simulink model "fwv_modified"  (R2021a)
settings: Solver=ode23t  StartTime=0.0  StopTime=9  FixedStep=0.01  MaxStep=0.01  RelTol=1e-3  AbsTol=1e-3  EnableMultiTasking=on
model workspace: external: MATLAB File param.m (data not in the file)
values from neighbouring files (symbols this model uses):
  A_D = 1.5    [main.m]    (also in param.m; params.m)
  A_L = 1.8    [main.m]    (also in param.m; params.m)
  c_bar = 0.035714285714285712    (= 0.0357142857143)    [main.m]    (also in param.m = 0.0251327412287; params.m)
  C_D0 = 0.45    [main.m]    (also in param.m; params.m)
  f = 37.5    [param.m]
  ht = 4    [main.m]    (also in param.m)
  m = 2    [rbf_pid.m]
  r00 = 0.93333333333333335    (= 0.933333333333)    [main.m]    (also in param.m = 1; params.m)
  r11 = 0.48118518518518516    (= 0.481185185185)    [main.m]    (also in param.m = double(int(curv(x)*(x+1/9),0,1)); params.m)
  r22 = 0.30475061728395064    (= 0.304750617284)    [main.m]    (also in param.m = double(int(curv(x)*(x+1/9)^2,0,1)); params.m)
  r33 = 0.2185686913580247    (= 0.218568691358)    [main.m]    (also in param.m = double(int(curv(x)*(x+1/9)^3,0,1)); params.m)
  r_cp = 0.10758076225045371    (= 0.10758076225)    [main.m]    (also in param.m = Rw*r33/r22; params.m)
  rho = 1.205    [main.m]    (also in param.m; params.m)
  Rw = 0.15    [main.m]    (also in param.m = 0.075; params.m)
  z00 = 1.0017777777777779    (= 1.00177777778)    [main.m]    (also in param.m = double(int(curv(x)^2,0,1)); params.m)
  z11 = 0.48491851851851853    (= 0.484918518519)    [main.m]    (also in param.m = double(int(curv(x)^2*(x+1/9),0,1)); params.m)
  z22 = 0.28785382716049385    (= 0.28785382716)    [main.m]    (also in param.m = double(int(curv(x)^2*(x+1/9)^2,0,1)); params.m)
  zrd = 1.2933386666666666    (= 1.29333866667)    [main.m]    (also in param.m = double(int(curv(x)^4,0,1)); params.m)
undefined symbols (not defined in the file or in its folder): X, Y, Z
libraries: sm_lib x63, nesl_utility x41, vrlib x3, slpidlib x2, simulink x1
(part 1 of 3)
settings Model: NumberOfSteps=10  PacingRate=1000  OrderedModelArguments=off  Creator=jeff  LastModifiedBy=jeff
settings SolverCC: AutoScaleAbsTol=off  ZeroCrossAlgorithm=Adaptive  SolverResetMethod=Robust
settings DataIOCC: LimitDataPoints=on  MaxDataPoints=10000  DSMLogging=off  InspectSignalLogs=on  SaveTime=off  ReturnWorkspaceOutputs=off
settings OptimizationCC: LifeSpan=inf
settings DebuggingCC: AllowSymbolicDim=off  SFUnexpectedBacktrackingDiag=warning  SFNoUnconditionalDefaultTransitionDiag=warning  SFExecutionAtInitializationDiag=none  SFMachineParentedDataDiag=warning  ArithmeticOperatorsInVariantConditions=warning
settings ModelReferenceCC: ModelReferenceMinAlgLoopOccurrences=on
settings SFSimCC: SimUseLocalCustomCode=off  CustomCodeUndefinedFunction=UseInterfaceOnly
settings RTWCC: RTWUseLocalCustomCode=off
settings CodeAppCC: StateflowObjectComments=on
settings GRTTargetCC: TargetLangStandard=C89/C90 (ANSI)
settings ConfigComp: CovMetricSettings=dw  CovSaveCumulativeToWorkspaceVar=on  CovSaveSingleToWorkspaceVar=on  CovExternalEMLEnable=off  CovSFcnEnable=off
settings SimscapeCC: SimscapeLogType=all  SimscapeLogSimulationStatistics=on  SimscapeLogDataHistory=10000
settings ExplorerConfigSet: InternalSimMechanicsExplorerSettings="<ExplorerConfiguration><canonicalview>default</canonicalview><AnimationSetting><BasePlaybackSpeed>1.0</BasePlaybackSpeed><PlaybackSpeedFactor>1.0</PlaybackSpeedFactor></AnimationSetting><TilePanel><TileInfo><Tiles Columns=\"2\" Count=\"4\" Rows=\"2\"><Column Weight=\"0.5\"/><Column Weight=\"0.5\"/><Row Weight=\"0.4982\"/><Row Weight=\"0.5018\"/><Tile Height=\"1\" Width=\"1\" X=\"0\" Y=\"0\"/><Tile Height=\"1\" Width=\"1\" X=\"0\" Y=\"1\"/><Tile Height=\"1\" Width=\"1\" X=\"1\" Y=\"0\"/><Tile Height=\"1\" Width=\"1\" X=\"1\" Y=\"1\"/></Tiles></TileInfo><SceneInfo><SceneViewer><BGColor><R>0.60000002384185791</R><G>0.60000002384185791</G><B>0.60000002384185791</B></BGColor><Camera><DoPerspective>off</DoPerspective><Position><X>1.52276591336431011e-07</X><Y>-15.7283506478538051</Y><Z>0.997276938595945239</Z></Position><Center><X>1.52276591336431011e-07</X><Y>8.81149515574719544e-08</Y><Z>0.997276938595945239</Z></Center><Up><X>0</X><Y>-0</Y><Z>1</Z></Up><ViewLimDist>1</ViewLimDist><YLim>4.13867069486404926</YLim><XLim>10.3000000000000007</XLim></Camera></SceneViewer><SceneViewer><BGColor><R>0.60000002384185791</R><G>0.60000002384185791</G><B>0.60000002384185791</B></BGColor><Camera><DoPerspective>off</DoPerspective><Position><X>1.52276591336431011e-07</X><Y>-4.72670020457144346e-07</Y><Z>14.1965844691727394</Z></Position><Center><X>1.52276591336431011e-07</X><Y>-4.72670020457144346e-07</Y><Z>0.997276770136494406</Z></Center><Up><X>0</X><Y>1</Y><Z>-0</Z></Up><ViewLimDist>1</ViewLimDist><YLim>10.3000000000000007</YLim><XLim>25.4425373134328368</XLim></Camera></SceneViewer><SceneViewer><BGColor><R>0.60000002384185791</R><G>0.60000002384185791</G><B>0.60000002384185791</B></BGColor><Camera><DoPerspective>off</DoPerspective><Position><X>15.7283506450403667</X><Y>-4.72670020457144346e-07</Y><Z>0.997277415433075021</Z></Position><Center><X>1.16597679067353965e-06</X><Y>-4.72670020457144346e-07</Y><Z>0.997277415433075021</Z></Center><Up><X>-0</X><Y>0</Y><Z>1</Z></Up><ViewLimDist>1</ViewLimDist><YLim>4.13867069486404926</YLim><XLim>10.3000000000000007</XLim></Camera></SceneViewer><SceneViewer><BGColor><R>0.60000002384185791</R><G>0.60000002384185791</G><B>0.60000002384185791</B></BGColor><Camera><DoPerspective>on</DoPerspective><Position><X>2.15185180954951205</X><Y>2.000061471445302</Y><Z>2.10008566610887026</Z></Position><Center><X>2.00185180954951214</X><Y>2.000061471445302</Y><Z>2.00008566610887017</Z></Center><Up><X>0</X><Y>-3.08148791101957736e-33</Y><Z>1</Z></Up><ViewLimDist>1</ViewLimDist><YLim>0.466307658154998583</YLim><XLim>1.15184951380078004</XLim></Camera></SceneViewer></SceneInfo></TilePanel><MechEditorPanel><Cameras><Camera><Id>Camera1</Id><Value><Name>Camera1</Name><NativeCamera><PositionTrackingFeature>FWV.camera.camera_Frame.R</PositionTrackingFeature><CenterTrackingFeature>FWV.camera.C</CenterTrackingFeature><UpVectorTrackingFeature>FWV.camera.C</UpVectorTrackingFeature><CenterTrackingOrigin>on</CenterTrackingOrigin><UpVectorTrackingDirection>+Z</UpVectorTrackingDirection></NativeCamera></Value></Camera></Cameras><GfxPanelCameraMap><MapElement CameraMLId=\"Camera1\" GfxPanelIndex=\"3\"/></GfxPanelCameraMap><VideoCreator><PlaybackSpeedRatio>1.0</PlaybackSpeedRatio><FrameRate>30</FrameRate><VideoFormat>Motion JPEG AVI</VideoFormat><FrameSize>auto</FrameSize></VideoCreator></MechEditorPanel></ExplorerConfiguration>"

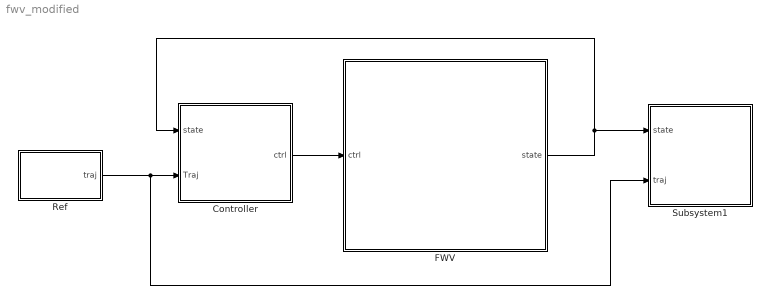
== system fwv_modified ==
  Controller : Subsystem
  FWV : Subsystem  mask{rho_w=800, m_t=20, stif_stk=1e-2, stif_rot=5e-3, damp_rot=0, stif_m=1e2, damp_m=1e2, z0=0, p0=0, q0=0, r0=0}
      mask prompts: z0 "initial height"; p0 "initial roll(deg)"; q0 "initial pitch(deg)"; r0 "initial yaw(deg)"
      mask Display: image('Images/fwv.png');
  Ref : Subsystem
  Subsystem1 : Subsystem
  wires:
  Ref/1(traj) -> Subsystem1/2(traj), Controller/2(Traj)
  Controller/1(ctrl) -> FWV/1(ctrl)
  FWV/1(state) -> Controller/1(state), Subsystem1/1(state)

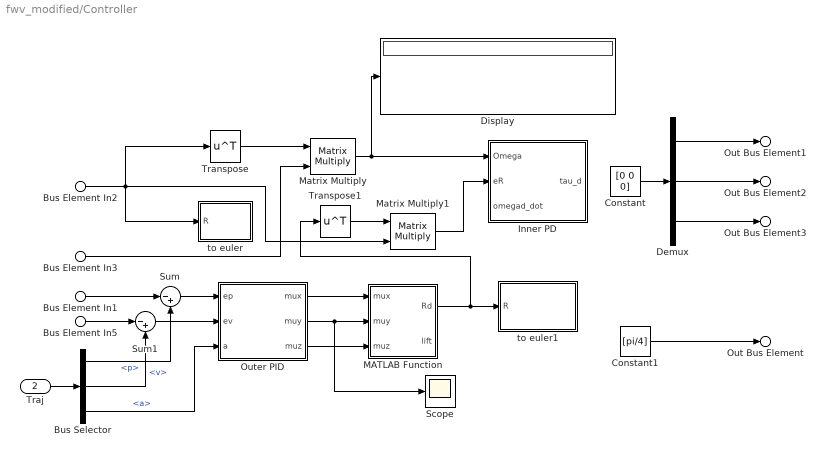
== system fwv_modified/Controller ==
  Bus Element In1 : Inport  PortName=state  Element=pose.p
  Bus Element In2 : Inport  PortName=state  Element=pose.R
  Bus Element In3 : Inport  PortName=state  Element=pose.Rd
  Bus Element In5 : Inport  PortName=state  Element=pose.v
  Traj : Inport  Port=2
  Bus Selector : BusSelector  OutputSignals=p,v,a
  Constant : Constant  Value=[0 0 0]
  Constant1 : Constant  Value=[pi/4]
  Demux : Demux  Outputs=3
  Display : Display
  Inner PD : Subsystem
  MATLAB Function : MATLAB Function  TreatAsAtomicUnit=on
  Matrix Multiply : Product  Multiplication=Matrix(*)
  Matrix Multiply1 : Product  Multiplication=Matrix(*)
  Outer PID : Subsystem
  Scope : Scope
  Sum : Sum  Inputs=|-+
  Sum1 : Sum  Inputs=|-+
  Transpose : Math  Operator=transpose  SaturateOnIntegerOverflow=on
  Transpose1 : Math  Operator=transpose  SaturateOnIntegerOverflow=on
  to euler : Subsystem
  to euler1 : Subsystem
  Out Bus Element : Outport  PortName=ctrl  Element=amp_mean
  Out Bus Element1 : Outport  PortName=ctrl  Element=amp_diff
  Out Bus Element2 : Outport  PortName=ctrl  Element=bias
  Out Bus Element3 : Outport  PortName=ctrl  Element=offset
  wires:
  Bus Element In1/1 -> Sum/1
  Traj/1 -> Bus Selector/1
  Bus Selector/1 -> Sum/2  "<p>"
  Demux/1 -> Out Bus Element1/1
  Demux/2 -> Out Bus Element2/1
  Demux/3 -> Out Bus Element3/1
  Bus Element In2/1 -> Matrix Multiply1/2, to euler/1(R), Transpose/1
  Sum/1 -> Outer PID/1(ep)
  Matrix Multiply1/1 -> Inner PD/2(eR)
  Matrix Multiply/1 -> Display/1, Inner PD/1(Omega)
  Transpose/1 -> Matrix Multiply/1
  Bus Element In3/1 -> Matrix Multiply/2
  Outer PID/1(mux) -> MATLAB Function/1(mux)
  Outer PID/2(muy) -> Scope/1, MATLAB Function/2(muy)
  Outer PID/3(muz) -> MATLAB Function/3(muz)
  Transpose1/1 -> Matrix Multiply1/1
  MATLAB Function/1(Rd) -> Transpose1/1, to euler1/1(R)
  Bus Element In5/1 -> Sum1/1
  Sum1/1 -> Outer PID/2(ev)
  Bus Selector/2 -> Sum1/2  "<v>"
  Bus Selector/3 -> Outer PID/3(a)  "<a>"
  Constant/1 -> Demux/1
  Constant1/1 -> Out Bus Element/1

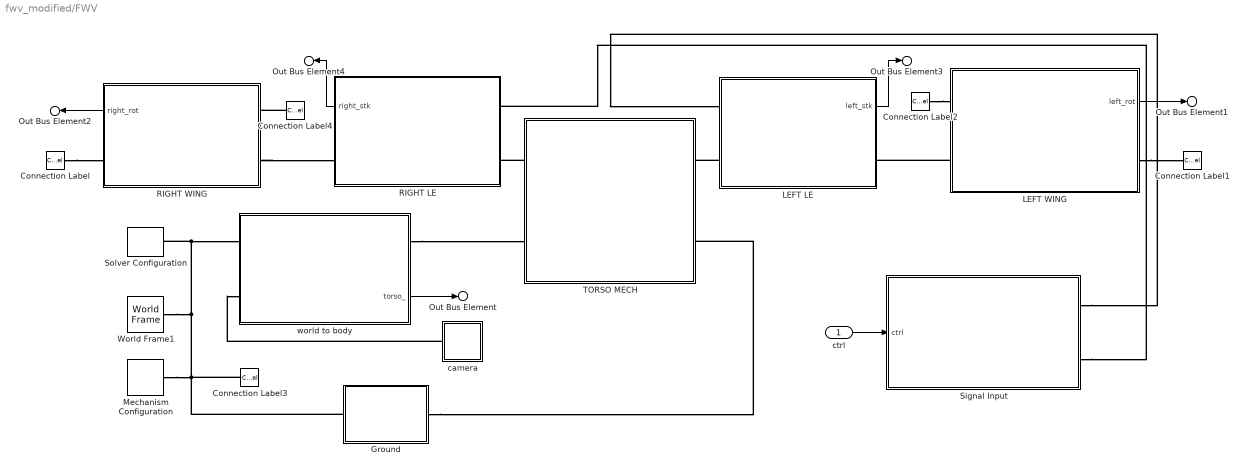
== system fwv_modified/FWV ==
  ctrl : Inport
  Connection Label : ConnectionLabel  Label=CP_R
  Connection Label1 : ConnectionLabel  Label=CP_L
  Connection Label2 : ConnectionLabel  Label=W
  Connection Label3 : ConnectionLabel  Label=W
  Connection Label4 : ConnectionLabel  Label=W
  Ground : Subsystem
  LEFT LE : Subsystem
      mask Display: image('Images/lle.png'); % Use "Edit Image" on toolstrip to change.
  LEFT WING : Subsystem
      mask Display: image('Images/lwing.png'); % Use "Edit Image" on toolstrip to change.
  Mechanism Configuration : sm_lib/Utilities/Mechanism Configuration  UniformGravity=Constant  GravityVector=[0 0 -9.80665]  GravityVectorUnits=m/s^2  GravityUnits=m/s^2  LinearizationDelta=0.001  JointModeTransitionNonlinearIterations=2
  RIGHT LE : Subsystem
      settings: PortSchema="{\"entries\":[{\"content\":{\"sides\":[{\"content\":{\"connectorIds\":[\"Out1\",\"LConn1\"]},\"type\":\"ConnectorPlacement.EquallySpacedRectSide\",\"uuid\":\"e80f0529-82a8-4e91-8f70-1f5fff48efb0\"},{\"content\":{\"connectorIds\":[\"RConn1\",\"RConn2\"],\"side\":\"RIGHT\"},\"type\":\"ConnectorPlacement.EquallySpacedRectSide\",\"uuid\":\"c7e3ee7d-7bee-46da-b210-768e5832b89d\"},{\"content\":{\"connectorIds\":[],\"side\":\"TOP\"},\"type\":\"ConnectorPlacement.EquallySpacedRectSide\",\"uuid\":\"680cbd67-40e5-4a58-a196-f2062cf587c7\"}]},\"type\":\"ConnectorPlacement.EquallySpacedConnector\",\"uuid\":\"7cb1a5ec-7352-40bf-9e6c-a29cba360f94\"}],\"packageUris\":[\"http://schema.mathworks.com/mf0/Connector/R2020b\"],\"version\":\"1.0\"}"
      mask Display: image('Images/rle.png'); % Use "Edit Image" on toolstrip to change.
  RIGHT WING : Subsystem
      mask Display: image('Images/rwing.png'); % Use "Edit Image" on toolstrip to change.
  Signal Input : Subsystem
  Solver Configuration : nesl_utility/Solver Configuration  PhysicalDomain=network_engine_domain  SubClassName=solver  LeftPortType=input  RightPortType=generic  Tones=[]  Harmonics=[]  SimulateNoise=off  Profile=off  UseLocalSampling=off  EnableSwitchedLinearOptims=on  FrequencyDomain=off  UseCCode=off  RelTol=0.001  AbsTol=1e-06  MinStep=1e-09  ToWorkspace=off  RevertToSquareIcSolve=off  NumHomotopyIterations=100  PhasorMode=off  PhasorModeNumHarmonics=1  DoDC=off  ResidualTolerance=1e-09  UseLocalSolver=off  LocalSolverChoice=NE_BACKWARD_EULER_ADVANCER  LocalSolverSampleTime=0.001  DoFixedCost=off  MaxNonlinIter=3  MaxModeIter=2  ComputeImpulses=off  ImpulseIterations=2  LinearAlgebra=Sparse  EquationFormulation=NE_TIME_EF  DelaysMemoryBudget=1024  AutomaticFiltering=on  FilteringTimeConstant=0.001  PartitionStorageMethod=AS_NEEDED  PartitionMemoryBudget=1024  PartitionMethod=FAST
      settings: SourceProductBaseCode=PW,SS
  TORSO MECH : Subsystem  mask{mu0=0, mu1=0}
      mask Display: image('Images/torso.png'); % Use "Edit Image" on toolstrip to change.
  World Frame1 : sm_lib/Frames and Transforms/World Frame
  camera : Subsystem
  world to body : Subsystem
      settings: PortSchema="{\"entries\":[{\"content\":{\"sides\":[{\"content\":{\"connectorIds\":[\"LConn1\",\"LConn2\"]},\"type\":\"ConnectorPlacement.EquallySpacedRectSide\",\"uuid\":\"67e08b7d-27a7-478e-aa2b-0a29cfb8c4ba\"},{\"content\":{\"connectorIds\":[\"RConn1\",\"Out1\"],\"side\":\"RIGHT\"},\"type\":\"ConnectorPlacement.EquallySpacedRectSide\",\"uuid\":\"af848fd7-c404-4734-a34f-7cffff1411b1\"},{\"content\":{\"connectorIds\":[],\"side\":\"TOP\"},\"type\":\"ConnectorPlacement.EquallySpacedRectSide\",\"uuid\":\"40c86437-2469-4d2e-8b61-7b3eee85e893\"}]},\"type\":\"ConnectorPlacement.EquallySpacedConnector\",\"uuid\":\"cd10b607-3f85-4cd2-a6c3-0d07bf2597bd\"}],\"packageUris\":[\"http://schema.mathworks.com/mf0/Connector/R2020b\"],\"version\":\"1.0\"}"
  Out Bus Element : Outport  PortName=state  Element=pose
  Out Bus Element3 : Outport  PortName=state  Element=left_stk
  Out Bus Element1 : Outport  PortName=state  Element=left_rot
  Out Bus Element4 : Outport  PortName=state  Element=right_stk
  Out Bus Element2 : Outport  PortName=state  Element=right_rot
  wires:
  LEFT WING/1(left_rot) -> Out Bus Element1/1
  RIGHT WING/1(right_rot) -> Out Bus Element2/1
  world to body/1(torso_) -> Out Bus Element/1
  ctrl/1 -> Signal Input/1(ctrl)
  LEFT LE/1(left_stk) -> Out Bus Element3/1
  RIGHT LE/1(right_stk) -> Out Bus Element4/1
  connections:
  LEFT LE/LConn2 -- TORSO MECH/RConn1
  TORSO MECH/LConn1 -- RIGHT LE/RConn2
  Mechanism Configuration/RConn1 -- Connection Label3/LConn1 -- Ground/LConn1 -- world to body/LConn1 -- Solver Configuration/RConn1 -- World Frame1/RConn1
  world to body/RConn1 -- TORSO MECH/LConn2
  camera/LConn1 -- world to body/LConn2
  Ground/RConn1 -- TORSO MECH/RConn2
  Connection Label/LConn1 -- RIGHT WING/RConn1
  LEFT WING/RConn1 -- Connection Label1/LConn1
  LEFT WING/LConn2 -- LEFT LE/RConn1
  RIGHT WING/LConn2 -- RIGHT LE/LConn1
  Connection Label2/LConn1 -- LEFT WING/LConn1
  Connection Label4/LConn1 -- RIGHT WING/LConn1
  Signal Input/RConn1 -- LEFT LE/LConn1
  Signal Input/RConn2 -- RIGHT LE/RConn1

== system fwv_modified/Ref ==
  Bus Creator : BusCreator  Inputs=3
  Clock : Clock
  Mux1 : Mux  Inputs=3
  p,pdot,pddot : MATLAB Function  TreatAsAtomicUnit=on
  pitch : Step  Time=0  After=2  SampleTime=0  ZeroCross=off
  roll : Step  Time=0  After=0  SampleTime=0  ZeroCross=off
  yaw : Step  Time=0  After=0  SampleTime=0  ZeroCross=off
  traj : Outport
  wires:
  roll/1 -> Mux1/1
  yaw/1 -> Mux1/3
  pitch/1 -> Mux1/2
  Bus Creator/1 -> traj/1
  p,pdot,pddot/2(v) -> Bus Creator/2  "v"
  p,pdot,pddot/3(a) -> Bus Creator/3  "a"
  Clock/1 -> p,pdot,pddot/1(t)
  p,pdot,pddot/1(p) -> Bus Creator/1  "p"

== system fwv_modified/Subsystem1 ==
  Bus Element In1 : Inport  PortName=state  Element=pose.p
  Bus Element In : Inport  Port=2  PortName=traj  Element=p
  Demux : Demux  Outputs=3
  Terminator : Terminator
  To Workspace : ToWorkspace  VariableName=p  SampleTime=-1
      settings: Save2DSignal=2-D array (concatenate along first dimension)
  To Workspace1 : ToWorkspace  VariableName=pd  SampleTime=-1
      settings: Save2DSignal=2-D array (concatenate along first dimension)
  XY Graph : simulink/Sinks/XY Graph  xmin=-2  xmax=1  ymin=-1  ymax=1  st=-1
  wires:
  Bus Element In1/1 -> To Workspace/1, Demux/1
  Demux/3 -> Terminator/1
  Demux/1 -> XY Graph/1
  Demux/2 -> XY Graph/2
  Bus Element In/1 -> To Workspace1/1

== system fwv_modified/Controller/Inner PD ==
  Omega : Inport
  eR : Inport  Port=2
  omegad_dot : Inport  Port=3
  Add : Sum  Inputs=-|-+
  Display : Display
  Display1 : Display
  Kd : Constant  Value=[d1,0,0;0,d2,0;0,0,d3]  mask{d1=0.02, d2=0.2, d3=0.02}
  Kp : Constant  Value=[p1,0,0;0,p2,0;0,0,p3]  mask{p1=0.3, p2=0.5, p3=0}
  Product : Product  Multiplication=Matrix(*)
  Product1 : Product  Multiplication=Matrix(*)
  Scope : Scope
  get D : Subsystem
  get P : Subsystem
  to euler1 : Subsystem
  tau_d : Outport
  wires:
  eR/1 -> to euler1/1(R), Display1/1, get P/1(eR)
  Omega/1 -> get D/1(In1)
  Kp/1 -> Product/1
  get P/1(Out) -> Product/2
  Add/1 -> tau_d/1
  Product1/1 -> Add/2
  Kd/1 -> Product1/1
  Product/1 -> Scope/1, Add/1
  get D/1(omega) -> Display/1, Product1/2
  omegad_dot/1 -> Add/3

== system fwv_modified/Controller/Outer PID ==
  ep : Inport
  ev : Inport  Port=2
  a : Inport  Port=3
  Demux : Demux  Outputs=3
  Demux1 : Demux  Outputs=3
  Demux2 : Demux  Outputs=3
  x PID : slpidlib/PID Controller  Commented=on  Controller=PID  Form=Parallel  TimeDomain=Continuous-time  UseExternalTs=off  SampleTime=-1  IntegratorMethod=Forward Euler  FilterMethod=Forward Euler  ControllerParametersSource=internal  P=0.5  I=0  D=0.1  UseFilter=on  N=25  TunerSelectOption=Transfer Function Based (PID Tuner App)  InitialConditionSource=internal  InitialConditionForIntegrator=0  InitialConditionForFilter=0  DifferentiatorICPrevScaledInput=0  ExternalReset=none  TrackingMode=off  Kt=1  LimitOutput=off  SatLimitsSource=internal  UpperSaturationLimit=0.5  LowerSaturationLimit=-0.5  LinearizeAsGain=on  AntiWindupMode=none  Kb=1  POutMin=[]  POutMax=[]  IOutMin=[]  IOutMax=[]  DOutMin=[]  DOutMax=[]  NOutMin=[]  NOutMax=[]  SumOutDataTypeStr=double  SumOutMin=[]  SumOutMax=[]  SaturationOutMin=[]  SaturationOutMax=[]  PParamMin=[]  PParamMax=[]  IParamMin=[]  IParamMax=[]  DParamMin=[]  DParamMax=[]  NParamMin=[]  NParamMax=[]  KbParamMin=[]  KbParamMax=[]  KtParamMin=[]  KtParamMax=[]  KbOutMin=[]  KbOutMax=[]  KtOutMin=[]  KtOutMax=[]  IntegratorOutMin=[]  IntegratorOutMax=[]  FilterOutMin=[]  FilterOutMax=[]  SumI1OutMin=[]  SumI1OutMax=[]  SumI2OutMin=[]  SumI2OutMax=[]  SumI3OutMin=[]  SumI3OutMax=[]  SumI4OutMin=[]  SumI4OutMax=[]  SumDOutMin=[]  SumDOutMax=[]  DifferentiatorOutMin=[]  DifferentiatorOutMax=[]  FilterDiffOutCoefMin=[]  FilterDiffOutCoefMax=[]  ReciprocalOutMin=[]  ReciprocalOutMax=[]  SumDenOutMin=[]  SumDenOutMax=[]  SumNumOutMin=[]  SumNumOutMax=[]  DivideOutMin=[]  DivideOutMax=[]  UdiffTsProdOutMin=[]  UdiffTsProdOutMax=[]  NTsProdOutMin=[]  NTsProdOutMax=[]  UintegralTsProdOutMin=[]  UintegralTsProdOutMax=[]  UngainTsProdOutMin=[]  UngainTsProdOutMax=[]  IntegratorContinuousStateAttributes=''  IntegratorStateMustResolveToSignalObject=off  IntegratorRTWStateStorageClass=Auto  FilterContinuousStateAttributes=''  FilterStateMustResolveToSignalObject=off  FilterRTWStateStorageClass=Auto  ParallelPVariant=InternalParameters  IdealPVariant=Disabled  IVariant=InternalParameters  DVariant=InternalParameters  IntegratorVariant=Continuous  SatVariant=Disabled  AWVariant=Passthrough  PCopyVariant=Disabled  TRVariant=Disabled  FdbkBlocksVariant=Forward  IdealPFdbkVariant=Disabled  SatFdbkVariant=Disabled  DerivativeFilterVariant=ContFilter  NVariant=InternalParameters  NCopyVariant=Disabled  FilterICVariant=InternalICsFilter  IntegratorICVariant=InternalICs  ExternalResetVariant=Disabled  TRSumVariant=Passthrough  SumFdbkVariant=Disabled  SumVariant=Sum_PID  TsampFilterVariant=InternalTs  TsampNgainVariant=Passthrough  TsampIntegralVariant=Passthrough  ExternalSaturationOutDataTypeStr=Inherit: Same as second input
  x PID1 : Subsystem  mask{Kp=0, Ki=0, Kd=0}
  y PID : slpidlib/PID Controller  Commented=on  Controller=PID  Form=Parallel  TimeDomain=Continuous-time  UseExternalTs=off  SampleTime=-1  IntegratorMethod=Forward Euler  FilterMethod=Forward Euler  ControllerParametersSource=internal  P=0.3  I=0  D=0.3  UseFilter=on  N=25  TunerSelectOption=Transfer Function Based (PID Tuner App)  InitialConditionSource=internal  InitialConditionForIntegrator=0  InitialConditionForFilter=0  DifferentiatorICPrevScaledInput=0  ExternalReset=none  TrackingMode=off  Kt=1  LimitOutput=off  SatLimitsSource=internal  UpperSaturationLimit=0.5  LowerSaturationLimit=-0.5  LinearizeAsGain=on  AntiWindupMode=none  Kb=1  POutMin=[]  POutMax=[]  IOutMin=[]  IOutMax=[]  DOutMin=[]  DOutMax=[]  NOutMin=[]  NOutMax=[]  SumOutMin=[]  SumOutMax=[]  SaturationOutMin=[]  SaturationOutMax=[]  PParamMin=[]  PParamMax=[]  IParamMin=[]  IParamMax=[]  DParamMin=[]  DParamMax=[]  NParamMin=[]  NParamMax=[]  KbParamMin=[]  KbParamMax=[]  KtParamMin=[]  KtParamMax=[]  KbOutMin=[]  KbOutMax=[]  KtOutMin=[]  KtOutMax=[]  IntegratorOutMin=[]  IntegratorOutMax=[]  FilterOutMin=[]  FilterOutMax=[]  SumI1OutMin=[]  SumI1OutMax=[]  SumI2OutMin=[]  SumI2OutMax=[]  SumI3OutMin=[]  SumI3OutMax=[]  SumI4OutMin=[]  SumI4OutMax=[]  SumDOutMin=[]  SumDOutMax=[]  DifferentiatorOutMin=[]  DifferentiatorOutMax=[]  FilterDiffOutCoefMin=[]  FilterDiffOutCoefMax=[]  ReciprocalOutMin=[]  ReciprocalOutMax=[]  SumDenOutMin=[]  SumDenOutMax=[]  SumNumOutMin=[]  SumNumOutMax=[]  DivideOutMin=[]  DivideOutMax=[]  UdiffTsProdOutMin=[]  UdiffTsProdOutMax=[]  NTsProdOutMin=[]  NTsProdOutMax=[]  UintegralTsProdOutMin=[]  UintegralTsProdOutMax=[]  UngainTsProdOutMin=[]  UngainTsProdOutMax=[]  IntegratorContinuousStateAttributes=''  IntegratorStateMustResolveToSignalObject=off  IntegratorRTWStateStorageClass=Auto  FilterContinuousStateAttributes=''  FilterStateMustResolveToSignalObject=off  FilterRTWStateStorageClass=Auto  ParallelPVariant=InternalParameters  IdealPVariant=Disabled  IVariant=InternalParameters  DVariant=InternalParameters  IntegratorVariant=Continuous  SatVariant=Disabled  AWVariant=Passthrough  PCopyVariant=Disabled  TRVariant=Disabled  FdbkBlocksVariant=Forward  IdealPFdbkVariant=Disabled  SatFdbkVariant=Disabled  DerivativeFilterVariant=ContFilter  NVariant=InternalParameters  NCopyVariant=Disabled  FilterICVariant=InternalICsFilter  IntegratorICVariant=InternalICs  ExternalResetVariant=Disabled  TRSumVariant=Passthrough  SumFdbkVariant=Disabled  SumVariant=Sum_PID  TsampFilterVariant=InternalTs  TsampNgainVariant=Passthrough  TsampIntegralVariant=Passthrough  ExternalSaturationOutDataTypeStr=Inherit: Same as second input
  y PID1 : Subsystem  mask{Kp=0, Ki=0, Kd=0}
  z PID1 : Subsystem  mask{Kp=50, Ki=40, Kd=20}
  mux : Outport
  muy : Outport  Port=2
  muz : Outport  Port=3
  wires:
  ep/1 -> Demux/1
  x PID1/1(Out1) -> mux/1
  y PID1/1(Out1) -> muy/1
  z PID1/1(Out1) -> muz/1
  a/1 -> Demux2/1
  Demux1/2 -> y PID1/2(In2)
  Demux2/3 -> z PID1/3(In3)
  Demux2/2 -> y PID1/3(In3)
  Demux1/1 -> x PID1/2(In2)
  Demux1/3 -> z PID1/2(In2)
  Demux/3 -> z PID1/1(In1)
  Demux2/1 -> x PID1/3(In3)
  Demux/1 -> x PID1/1(In1)
  Demux/2 -> y PID1/1(In1)
  ev/1 -> Demux1/1

== system fwv_modified/Controller/to euler ==
  R : Inport
  Mux : Mux  Inputs=3
  R to X-Y-Z Extrinsic : Subsystem  mask(Rotation Matrix to X-Y-Z Extrinsic){}
      mask help: Computes roll / pitch / yaw values assuming they correspond to X, Y, and Z rotations, applied in that order and using extrinsic rotations (rotations applied about the fixed axes of the base frame). Does not handle case where Y (pitch) rotation is +/-90 degrees.
  Terminator : Terminator
  rad2deg : Gain  Gain=180/pi
  wires:
  R/1 -> R to X-Y-Z Extrinsic/1(R)
  R to X-Y-Z Extrinsic/2(pitch) -> Mux/2
  Mux/1 -> rad2deg/1
  rad2deg/1 -> Terminator/1
  R to X-Y-Z Extrinsic/1(roll) -> Mux/1
  R to X-Y-Z Extrinsic/3(yaw) -> Mux/3

== system fwv_modified/Controller/to euler1 ==
  R : Inport
  Mux : Mux  Inputs=3
  R to X-Y-Z Extrinsic : Subsystem  mask(Rotation Matrix to X-Y-Z Extrinsic){}
      mask help: Computes roll / pitch / yaw values assuming they correspond to X, Y, and Z rotations, applied in that order and using extrinsic rotations (rotations applied about the fixed axes of the base frame). Does not handle case where Y (pitch) rotation is +/-90 degrees.
  Terminator : Terminator
  rad2deg : Gain  Gain=180/pi
  wires:
  rad2deg/1 -> Terminator/1
  R/1 -> R to X-Y-Z Extrinsic/1(R)
  Mux/1 -> rad2deg/1
  R to X-Y-Z Extrinsic/3(yaw) -> Mux/3
  R to X-Y-Z Extrinsic/1(roll) -> Mux/1
  R to X-Y-Z Extrinsic/2(pitch) -> Mux/2

== system fwv_modified/FWV/Ground ==
  Cylindrical Solid : sm_lib/Body Elements/Cylindrical Solid  GraphicAmbientColor=[0.15 0.15 0.15 1.0]  BasedOnType=Mass  CenterOfMass=[0 0 0]  CenterOfMassUnits=m  GraphicDiffuseColor=[1.0 0.2 0.4]  CylinderLength=1  CylinderLengthUnits=mm  CylinderRadius=10  CylinderRadiusUnits=m  Density=1000  DensityUnits=kg/m^3  DoExposeReferenceFrame=off  GraphicEmissiveColor=[0.0 0.0 0.0 1.0]  ExportEntireGeometry=on  SerializedFrames=<Frames><Frame><Id>Frame1</Id><Value><Name>F1</Name><Origin><Source>GeometricFeature</Source><FeatureName>top surface</FeatureName></Origin><PrimaryAxis><DefinedDirection>+Z</DefinedDirection><Source>ReferenceFrame</Source><SourceDirection>+Z</SourceDirection><FeatureName></FeatureName></PrimaryAxis><SecondaryAxis><DefinedDirection>+X</DefinedDirection><Source>ReferenceFrame</Source><SourceDirection>+X</SourceDirection><FeatureName></FeatureName></SecondaryAxis></Value></Frame></Frames>  MarkerShape=Sphere  MarkerSize=10  GraphicType=FromGeometry  InertiaType=Custom  Mass=0  MassUnits=kg  MomentsOfInertia=[1 1 1]  MomentsOfInertiaUnits=kg*m^2  GraphicOpacity=1.0  ProductsOfInertia=[0 0 0]  ProductsOfInertiaUnits=kg*m^2  GraphicShininess=75  GraphicSpecularColor=[0.5 0.5 0.5 1.0]  GraphicVisPropType=SimpleVisualProperties
  Rigid Transform : sm_lib/Frames and Transforms/Rigid Transform  TranslationMethod=StandardAxis  TranslationStandardOffset=5  TranslationLengthUnit=cm  TranslationStandardAxis=-Z  TranslationCartesianOffset=[0 0 0]  TranslationROffset=0  TranslationROffsetUnits=m  TranslationZOffset=0  TranslationZOffsetUnits=m  TranslationThetaOffset=0  TranslationThetaOffsetUnits=deg  RotationMethod=None  RotationAngleUnits=deg  RotationStandardAxis=+Z  RotationAngle=0.0  RotationArbitraryAxis=[0 0 1]  FollAlignAxisA=+X  BaseAlignAxisA=+Y  FollAlignAxisB=+Y  BaseAlignAxisB=+Z  RotationSequenceAxes=FollowerAxes  RotationSequence=XYX  RotationSequenceAngles=[0 0 0]  RotationSequenceAnglesUnits=deg  RotationMatrix=[1 0 0; 0 1 0; 0 0 1]
  W : PMIOPort  Side=Left
  G : PMIOPort  Port=2  Side=Right
  connections:
  G/RConn1 -- Cylindrical Solid/RConn1
  Rigid Transform/LConn1 -- W/RConn1
  Rigid Transform/RConn1 -- Cylindrical Solid/LConn1

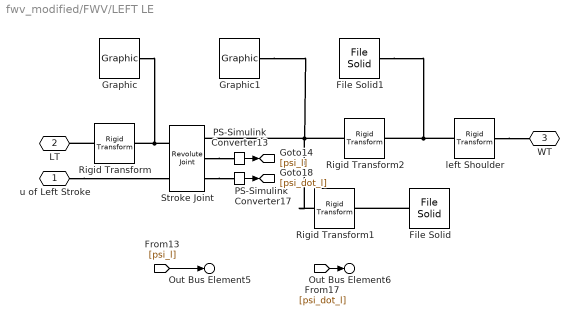
== system fwv_modified/FWV/LEFT LE ==
  File Solid : sm_lib/Body Elements/File Solid  ExtGeomFileName=/home/jeff/文档/research/fwvlab/meshes/ulna_radius.STL  UnitType=Custom  ExtGeomFileUnits=m  StepReaderType=HEX  ExportConvexHullGeometry=off  InertiaType=CalculateFromGeometry  Mass=1  MassUnits=kg  CenterOfMass=[0 0 0]  CenterOfMassUnits=m  MomentsOfInertia=[1 1 1]  MomentsOfInertiaUnits=kg*m^2  ProductsOfInertia=[0 0 0]  ProductsOfInertiaUnits=kg*m^2  BasedOnType=Density  Density=3500  DensityUnits=kg/m^3  DoExposeReferenceFrame=off  SerializedFrames=<Frames><Frame><Id>Frame1</Id><Value><Name>R</Name><Origin><Source>CenterOfMassFrame</Source><FeatureName></FeatureName></Origin><PrimaryAxis><DefinedDirection>+Z</DefinedDirection><Source>ReferenceFrame</Source><SourceDirection>+Z</SourceDirection><FeatureName></FeatureName></PrimaryAxis><SecondaryAxis><DefinedDirection>-Y</DefinedDirection><Source>ReferenceFrame</Source><SourceDirection>+X</SourceDirection><FeatureName></FeatureName></SecondaryAxis></Value></Frame></Frames>  GraphicType=FromGeometry  MarkerShape=Sphere  MarkerSize=10  GraphicVisPropType=SimpleVisualProperties  GraphicDiffuseColor=[0.5 0.5 0.5]  GraphicSpecularColor=[0.5 0.5 0.5 1.0]  GraphicAmbientColor=[0.15 0.15 0.15 1.0]  GraphicEmissiveColor=[0.0 0.0 0.0 1.0]  GraphicShininess=75  GraphicOpacity=1.0
  File Solid1 : sm_lib/Body Elements/File Solid  ExtGeomFileName=/home/jeff/文档/research/fwvlab/meshes/wingF - manus-1.STL  UnitType=Custom  ExtGeomFileUnits=mm  StepReaderType=HEX  ExportConvexHullGeometry=off  InertiaType=CalculateFromGeometry  Mass=1  MassUnits=kg  CenterOfMass=[0 0 0]  CenterOfMassUnits=m  MomentsOfInertia=[1 1 1]  MomentsOfInertiaUnits=kg*m^2  ProductsOfInertia=[0 0 0]  ProductsOfInertiaUnits=kg*m^2  BasedOnType=Density  Density=3500  DensityUnits=kg/m^3  DoExposeReferenceFrame=off  SerializedFrames=<Frames><Frame><Id>Frame2</Id><Value><Name>R</Name><Origin><Source>CenterOfMassFrame</Source><FeatureName></FeatureName></Origin><PrimaryAxis><DefinedDirection>+Z</DefinedDirection><Source>ReferenceFrame</Source><SourceDirection>+Z</SourceDirection><FeatureName></FeatureName></PrimaryAxis><SecondaryAxis><DefinedDirection>+Y</DefinedDirection><Source>ReferenceFrame</Source><SourceDirection>+X</SourceDirection><FeatureName></FeatureName></SecondaryAxis></Value></Frame></Frames>  GraphicType=FromGeometry  MarkerShape=Sphere  MarkerSize=10  GraphicVisPropType=SimpleVisualProperties  GraphicDiffuseColor=[0.5 0.5 0.5]  GraphicSpecularColor=[0.5 0.5 0.5 1.0]  GraphicAmbientColor=[0.15 0.15 0.15 1.0]  GraphicEmissiveColor=[0.0 0.0 0.0 1.0]  GraphicShininess=75  GraphicOpacity=1.0
  Graphic : sm_lib/Body Elements/Graphic  GraphicType=Marker  MarkerShape=Frame  MarkerSize=10  GraphicVisPropType=SimpleVisualProperties  GraphicDiffuseColor=[1.0 0.4 0.4]  GraphicSpecularColor=[0.5 0.5 0.5 1.0]  GraphicAmbientColor=[0.15 0.15 0.15 1.0]  GraphicEmissiveColor=[0.0 0.0 0.0 1.0]  GraphicShininess=75  GraphicOpacity=1.0
  Graphic1 : sm_lib/Body Elements/Graphic  GraphicType=Marker  MarkerShape=Frame  MarkerSize=10  GraphicVisPropType=SimpleVisualProperties  GraphicDiffuseColor=[0.2 0.2 1.0]  GraphicSpecularColor=[0.5 0.5 0.5 1.0]  GraphicAmbientColor=[0.15 0.15 0.15 1.0]  GraphicEmissiveColor=[0.0 0.0 0.0 1.0]  GraphicShininess=75  GraphicOpacity=1.0
  PS-Simulink Converter13 : nesl_utility/PS-Simulink Converter  PhysicalDomain=network_engine_domain  SubClassName=ps_output  LeftPortType=input  RightPortType=output  PseudoPeriodic=off  Frequencies=[]  Unit=inherit  AffineConversion=off
      settings: SourceProductBaseCode=PW,SS
  PS-Simulink Converter17 : nesl_utility/PS-Simulink Converter  PhysicalDomain=network_engine_domain  SubClassName=ps_output  LeftPortType=input  RightPortType=output  PseudoPeriodic=off  Frequencies=[]  Unit=inherit  AffineConversion=off
      settings: SourceProductBaseCode=PW,SS
  Rigid Transform : sm_lib/Frames and Transforms/Rigid Transform  TranslationMethod=StandardAxis  TranslationStandardOffset=0.18  TranslationLengthUnit=cm  TranslationStandardAxis=+Y  TranslationCartesianOffset=[0 0 0]  TranslationROffset=0  TranslationROffsetUnits=m  TranslationZOffset=0  TranslationZOffsetUnits=m  TranslationThetaOffset=0  TranslationThetaOffsetUnits=deg  RotationMethod=None  RotationAngleUnits=deg  RotationStandardAxis=+Z  RotationAngle=0.0  RotationArbitraryAxis=[0 0 1]  FollAlignAxisA=+X  BaseAlignAxisA=+Y  FollAlignAxisB=+Y  BaseAlignAxisB=+Z  RotationSequenceAxes=FollowerAxes  RotationSequence=XYX  RotationSequenceAngles=[0 0 0]  RotationSequenceAnglesUnits=deg  RotationMatrix=[1 0 0; 0 1 0; 0 0 1]
  Rigid Transform1 : sm_lib/Frames and Transforms/Rigid Transform  TranslationMethod=StandardAxis  TranslationStandardOffset=0.18  TranslationLengthUnit=cm  TranslationStandardAxis=+Y  TranslationCartesianOffset=[0 0 0]  TranslationROffset=0  TranslationROffsetUnits=m  TranslationZOffset=0  TranslationZOffsetUnits=m  TranslationThetaOffset=0  TranslationThetaOffsetUnits=deg  RotationMethod=None  RotationAngleUnits=deg  RotationStandardAxis=+Z  RotationAngle=0.0  RotationArbitraryAxis=[0 0 1]  FollAlignAxisA=+X  BaseAlignAxisA=+Y  FollAlignAxisB=+Y  BaseAlignAxisB=+Z  RotationSequenceAxes=FollowerAxes  RotationSequence=XYX  RotationSequenceAngles=[0 0 0]  RotationSequenceAnglesUnits=deg  RotationMatrix=[1 0 0; 0 1 0; 0 0 1]
  Rigid Transform2 : sm_lib/Frames and Transforms/Rigid Transform  TranslationMethod=StandardAxis  TranslationStandardOffset=1  TranslationLengthUnit=cm  TranslationStandardAxis=+Y  TranslationCartesianOffset=[0 0 0]  TranslationROffset=0  TranslationROffsetUnits=m  TranslationZOffset=0  TranslationZOffsetUnits=m  TranslationThetaOffset=0  TranslationThetaOffsetUnits=deg  RotationMethod=None  RotationAngleUnits=deg  RotationStandardAxis=+Z  RotationAngle=0.0  RotationArbitraryAxis=[0 0 1]  FollAlignAxisA=+X  BaseAlignAxisA=+Y  FollAlignAxisB=+Y  BaseAlignAxisB=+Z  RotationSequenceAxes=FollowerAxes  RotationSequence=XYX  RotationSequenceAngles=[0 0 0]  RotationSequenceAnglesUnits=deg  RotationMatrix=[1 0 0; 0 1 0; 0 0 1]
  Stroke Joint : sm_lib/Joints/Revolute Joint  JointMode=Normal  SenseConstraintForce=off  SenseConstraintForceX=off  SenseConstraintForceY=off  SenseConstraintForceZ=off  SenseConstraintTorque=off  SenseConstraintTorqueX=off  SenseConstraintTorqueY=off  SenseConstraintTorqueZ=off  SenseTotalForce=off  SenseTotalForceX=off  SenseTotalForceY=off  SenseTotalForceZ=off  SenseTotalTorque=off  SenseTotalTorqueX=off  SenseTotalTorqueY=off  SenseTotalTorqueZ=off  CompositeWrenchDir=FollowerOnBase  CompositeWrenchFrame=BaseFrame  EquilibriumPosition=0  EquilibriumPositionUnits=deg  SpringStiffness=stif_stk  SpringStiffnessUnits=N*m/rad  DampingCoefficient=0  DampingCoefficientUnits=N*m/(rad/s)  TorqueActuationMode=ComputedTorque  MotionActuationMode=InputMotion  SensePosition=on  SenseVelocity=on  SenseAcceleration=off  SenseTorqueForce=off  SenseLowerLimitTorqueForce=off  SenseUpperLimitTorqueForce=off  LowerLimitSpecify=on  LowerLimitBound=-90  LowerLimitBoundUnits=deg  LowerLimitStiffness=1e6  LowerLimitStiffnessUnits=N*m/rad  LowerLimitDamping=1e3  LowerLimitDampingUnits=N*m/(rad/s)  LowerLimitTransitionRegionWidth=0.1  LowerLimitTransitionRegionWidthUnits=deg  UpperLimitSpecify=on  UpperLimitBound=90  UpperLimitBoundUnits=deg  UpperLimitStiffness=1e6  UpperLimitStiffnessUnits=N*m/rad  UpperLimitDamping=1e3  UpperLimitDampingUnits=N*m/(rad/s)  UpperLimitTransitionRegionWidth=0.1  UpperLimitTransitionRegionWidthUnits=deg  PositionTargetSpecify=on  PositionTargetPriority=High  PositionTargetValue=-30  PositionTargetValueUnits=deg  VelocityTargetSpecify=off  VelocityTargetPriority=High  VelocityTargetValue=0  VelocityTargetValueUnits=deg/s
  left Shoulder : sm_lib/Frames and Transforms/Rigid Transform  TranslationMethod=Cartesian  TranslationStandardOffset=0  TranslationLengthUnit=cm  TranslationStandardAxis=+Z  TranslationCartesianOffset=[0 -0.25 0]  TranslationROffset=0  TranslationROffsetUnits=m  TranslationZOffset=0  TranslationZOffsetUnits=m  TranslationThetaOffset=0  TranslationThetaOffsetUnits=deg  RotationMethod=StandardAxis  RotationAngleUnits=deg  RotationStandardAxis=+X  RotationAngle=-90  RotationArbitraryAxis=[0 0 1]  FollAlignAxisA=+X  BaseAlignAxisA=+Y  FollAlignAxisB=+Y  BaseAlignAxisB=+Z  RotationSequenceAxes=FollowerAxes  RotationSequence=XYX  RotationSequenceAngles=[0 0 0]  RotationSequenceAnglesUnits=deg  RotationMatrix=[0 1 0; 0 0 1; 1 0 0]
  u of Left Stroke : PMIOPort  Side=Left
  LT : PMIOPort  Port=2  Side=Left
  WT : PMIOPort  Port=3  Side=Right
  Out Bus Element5 : Outport  PortName=left_stk  Element=q
  Out Bus Element6 : Outport  PortName=left_stk  Element=w
  wires:
  PS-Simulink Converter17/1 -> [psi_dot_l]
  PS-Simulink Converter13/1 -> [psi_l]
  [psi_l] -> Out Bus Element5/1
  [psi_dot_l] -> Out Bus Element6/1
  connections:
  Stroke Joint/RConn3 -- PS-Simulink Converter17/LConn1
  Stroke Joint/RConn2 -- PS-Simulink Converter13/LConn1
  Stroke Joint/LConn1 -- Graphic/RConn1 -- Rigid Transform/RConn1
  File Solid1/LConn1 -- left Shoulder/LConn1 -- Rigid Transform2/RConn1
  u of Left Stroke/RConn1 -- Stroke Joint/LConn2
  Rigid Transform/LConn1 -- LT/RConn1
  File Solid/LConn1 -- Rigid Transform1/RConn1
  left Shoulder/RConn1 -- WT/RConn1
  Rigid Transform2/LConn1 -- Rigid Transform1/LConn1 -- Stroke Joint/RConn1 -- Graphic1/RConn1

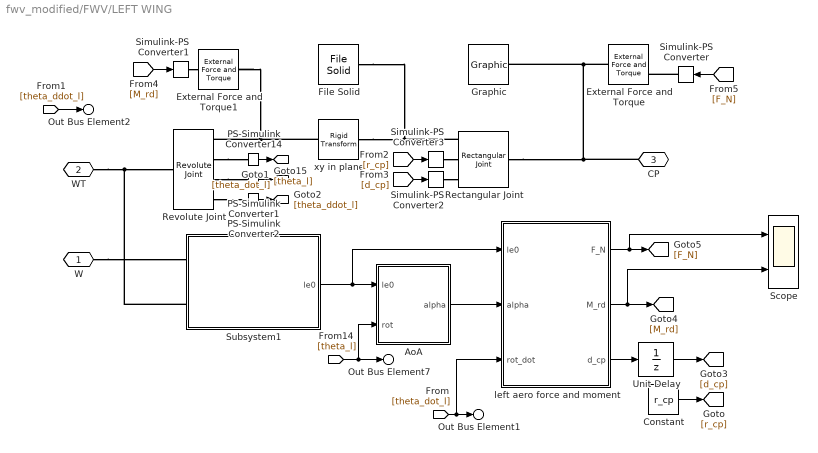
== system fwv_modified/FWV/LEFT WING ==
  AoA : MATLAB Function  TreatAsAtomicUnit=on
  Constant : Constant  Value=r_cp
  External Force and Torque : sm_lib/Forces and Torques/External Force and Torque  ForceResolutionFrame=AttachedFrame  EnableForceX=off  EnableForceY=on  EnableForceZ=on  EnableForce=off  TorqueResolutionFrame=AttachedFrame  EnableTorqueX=off  EnableTorqueY=off  EnableTorqueZ=off  EnableTorque=off
  External Force and Torque1 : sm_lib/Forces and Torques/External Force and Torque  ForceResolutionFrame=AttachedFrame  EnableForceX=off  EnableForceY=off  EnableForceZ=off  EnableForce=off  TorqueResolutionFrame=AttachedFrame  EnableTorqueX=off  EnableTorqueY=off  EnableTorqueZ=on  EnableTorque=off
  File Solid : sm_lib/Body Elements/File Solid  ExtGeomFileName=/home/jeff/文档/research/fwvlab/meshes/left_Wing.step  UnitType=Custom  ExtGeomFileUnits=mm  StepReaderType=HEX  ExportConvexHullGeometry=off  InertiaType=CalculateFromGeometry  Mass=1  MassUnits=kg  CenterOfMass=[0 0 0]  CenterOfMassUnits=m  MomentsOfInertia=[1 1 1]  MomentsOfInertiaUnits=kg*m^2  ProductsOfInertia=[0 0 0]  ProductsOfInertiaUnits=kg*m^2  BasedOnType=Density  Density=600  DensityUnits=kg/m^3  DoExposeReferenceFrame=on  SerializedFrames=<Frames/>  GraphicType=FromGeometry  MarkerShape=Sphere  MarkerSize=10  GraphicVisPropType=SimpleVisualProperties  GraphicDiffuseColor=[0.5 0.5 0.5]  GraphicSpecularColor=[0.5 0.5 0.5 1.0]  GraphicAmbientColor=[0.15 0.15 0.15 1.0]  GraphicEmissiveColor=[0.0 0.0 0.0 1.0]  GraphicShininess=75  GraphicOpacity=1.0
  Graphic : sm_lib/Body Elements/Graphic  GraphicType=Marker  MarkerShape=Frame  MarkerSize=20  GraphicVisPropType=SimpleVisualProperties  GraphicDiffuseColor=[1 0 1]  GraphicSpecularColor=[0.5 0.5 0.5 1.0]  GraphicAmbientColor=[0.15 0.15 0.15 1.0]  GraphicEmissiveColor=[0.0 0.0 0.0 1.0]  GraphicShininess=75  GraphicOpacity=1.0
  PS-Simulink Converter1 : nesl_utility/PS-Simulink Converter  PhysicalDomain=network_engine_domain  SubClassName=ps_output  LeftPortType=input  RightPortType=output  PseudoPeriodic=off  Frequencies=[]  Unit=inherit  AffineConversion=off
      settings: SourceProductBaseCode=PW,SS
  PS-Simulink Converter14 : nesl_utility/PS-Simulink Converter  PhysicalDomain=network_engine_domain  SubClassName=ps_output  LeftPortType=input  RightPortType=output  PseudoPeriodic=off  Frequencies=[]  Unit=inherit  AffineConversion=off
      settings: SourceProductBaseCode=PW,SS
  PS-Simulink Converter2 : nesl_utility/PS-Simulink Converter  PhysicalDomain=network_engine_domain  SubClassName=ps_output  LeftPortType=input  RightPortType=output  PseudoPeriodic=off  Frequencies=[]  Unit=inherit  AffineConversion=off
      settings: SourceProductBaseCode=PW,SS
  Rectangular Joint : sm_lib/Joints/Rectangular Joint  JointMode=Normal  SenseConstraintForce=off  SenseConstraintForceX=off  SenseConstraintForceY=off  SenseConstraintForceZ=off  SenseConstraintTorque=off  SenseConstraintTorqueX=off  SenseConstraintTorqueY=off  SenseConstraintTorqueZ=off  SenseTotalForce=off  SenseTotalForceX=off  SenseTotalForceY=off  SenseTotalForceZ=off  SenseTotalTorque=off  SenseTotalTorqueX=off  SenseTotalTorqueY=off  SenseTotalTorqueZ=off  CompositeWrenchDir=FollowerOnBase  CompositeWrenchFrame=BaseFrame  PxEquilibriumPosition=0  PxEquilibriumPositionUnits=m  PxSpringStiffness=0  PxSpringStiffnessUnits=N/m  PxDampingCoefficient=0  PxDampingCoefficientUnits=N/(m/s)  PxTorqueActuationMode=ComputedTorque  PxMotionActuationMode=InputMotion  PxSensePosition=off  PxSenseVelocity=off  PxSenseAcceleration=off  PxSenseTorqueForce=off  PxSenseLowerLimitTorqueForce=off  PxSenseUpperLimitTorqueForce=off  PxLowerLimitSpecify=off  PxLowerLimitBound=-1  PxLowerLimitBoundUnits=m  PxLowerLimitStiffness=1e6  PxLowerLimitStiffnessUnits=N/m  PxLowerLimitDamping=1e3  PxLowerLimitDampingUnits=N/(m/s)  PxLowerLimitTransitionRegionWidth=1e-4  PxLowerLimitTransitionRegionWidthUnits=m  PxUpperLimitSpecify=off  PxUpperLimitBound=1  PxUpperLimitBoundUnits=m  PxUpperLimitStiffness=1e6  PxUpperLimitStiffnessUnits=N/m  PxUpperLimitDamping=1e3  PxUpperLimitDampingUnits=N/(m/s)  PxUpperLimitTransitionRegionWidth=1e-4  PxUpperLimitTransitionRegionWidthUnits=m  PxPositionTargetSpecify=off  PxPositionTargetPriority=High  PxPositionTargetValue=0  PxPositionTargetValueUnits=m  PxVelocityTargetSpecify=off  PxVelocityTargetPriority=High  PxVelocityTargetValue=0  PxVelocityTargetValueUnits=m/s  PyEquilibriumPosition=0  PyEquilibriumPositionUnits=m  PySpringStiffness=0  PySpringStiffnessUnits=N/m  PyDampingCoefficient=0  PyDampingCoefficientUnits=N/(m/s)  PyTorqueActuationMode=ComputedTorque  PyMotionActuationMode=InputMotion  PySensePosition=off  PySenseVelocity=off  PySenseAcceleration=off  PySenseTorqueForce=off  PySenseLowerLimitTorqueForce=off  PySenseUpperLimitTorqueForce=off  PyLowerLimitSpecify=off  PyLowerLimitBound=-1  PyLowerLimitBoundUnits=m  PyLowerLimitStiffness=1e6  PyLowerLimitStiffnessUnits=N/m  PyLowerLimitDamping=1e3  PyLowerLimitDampingUnits=N/(m/s)  PyLowerLimitTransitionRegionWidth=1e-4  PyLowerLimitTransitionRegionWidthUnits=m  PyUpperLimitSpecify=off  PyUpperLimitBound=1  PyUpperLimitBoundUnits=m  PyUpperLimitStiffness=1e6  PyUpperLimitStiffnessUnits=N/m  PyUpperLimitDamping=1e3  PyUpperLimitDampingUnits=N/(m/s)  PyUpperLimitTransitionRegionWidth=1e-4  PyUpperLimitTransitionRegionWidthUnits=m  PyPositionTargetSpecify=off  PyPositionTargetPriority=High  PyPositionTargetValue=0  PyPositionTargetValueUnits=m  PyVelocityTargetSpecify=off  PyVelocityTargetPriority=High  PyVelocityTargetValue=0  PyVelocityTargetValueUnits=m/s
  Revolute Joint : sm_lib/Joints/Revolute Joint  JointMode=Normal  SenseConstraintForce=off  SenseConstraintForceX=off  SenseConstraintForceY=off  SenseConstraintForceZ=off  SenseConstraintTorque=off  SenseConstraintTorqueX=off  SenseConstraintTorqueY=off  SenseConstraintTorqueZ=off  SenseTotalForce=off  SenseTotalForceX=off  SenseTotalForceY=off  SenseTotalForceZ=off  SenseTotalTorque=off  SenseTotalTorqueX=off  SenseTotalTorqueY=off  SenseTotalTorqueZ=off  CompositeWrenchDir=FollowerOnBase  CompositeWrenchFrame=BaseFrame  EquilibriumPosition=0  EquilibriumPositionUnits=deg  SpringStiffness=stif_rot  SpringStiffnessUnits=N*m/rad  DampingCoefficient=damp_rot  DampingCoefficientUnits=N*m/(rad/s)  TorqueActuationMode=NoTorque  MotionActuationMode=ComputedMotion  SensePosition=on  SenseVelocity=on  SenseAcceleration=on  SenseTorqueForce=off  SenseLowerLimitTorqueForce=off  SenseUpperLimitTorqueForce=off  LowerLimitSpecify=on  LowerLimitBound=-45  LowerLimitBoundUnits=deg  LowerLimitStiffness=stif_m  LowerLimitStiffnessUnits=N*m/rad  LowerLimitDamping=damp_m  LowerLimitDampingUnits=N*m/(rad/s)  LowerLimitTransitionRegionWidth=0.1  LowerLimitTransitionRegionWidthUnits=deg  UpperLimitSpecify=on  UpperLimitBound=45  UpperLimitBoundUnits=deg  UpperLimitStiffness=stif_m  UpperLimitStiffnessUnits=N*m/rad  UpperLimitDamping=damp_m  UpperLimitDampingUnits=N*m/(rad/s)  UpperLimitTransitionRegionWidth=0.1  UpperLimitTransitionRegionWidthUnits=deg  PositionTargetSpecify=off  PositionTargetPriority=High  PositionTargetValue=20  PositionTargetValueUnits=deg  VelocityTargetSpecify=off  VelocityTargetPriority=High  VelocityTargetValue=0  VelocityTargetValueUnits=deg/s
  Scope : Scope  NumInputPorts=2
  Simulink-PS Converter : nesl_utility/Simulink-PS Converter  PhysicalDomain=network_engine_domain  SubClassName=ps_input  LeftPortType=input  RightPortType=output  PseudoPeriodic=off  Frequencies=[]  NoiseDistribution=none  NoiseParameters=[]  Unit=1  AffineConversion=off  FilteringAndDerivatives=provide  SimscapeFilterOrder=1  InputFilterTimeConstant=0.001  UdotUserProvided=0
      settings: SourceProductBaseCode=PW,SS
  Simulink-PS Converter1 : nesl_utility/Simulink-PS Converter  PhysicalDomain=network_engine_domain  SubClassName=ps_input  LeftPortType=input  RightPortType=output  PseudoPeriodic=off  Frequencies=[]  NoiseDistribution=none  NoiseParameters=[]  Unit=1  AffineConversion=off  FilteringAndDerivatives=provide  SimscapeFilterOrder=1  InputFilterTimeConstant=0.001  UdotUserProvided=0
      settings: SourceProductBaseCode=PW,SS
  Simulink-PS Converter2 : nesl_utility/Simulink-PS Converter  PhysicalDomain=network_engine_domain  SubClassName=ps_input  LeftPortType=input  RightPortType=output  PseudoPeriodic=off  Frequencies=[]  NoiseDistribution=none  NoiseParameters=[]  Unit=1  AffineConversion=off  FilteringAndDerivatives=filter  SimscapeFilterOrder=2  InputFilterTimeConstant=0.001  UdotUserProvided=0
      settings: SourceProductBaseCode=PW,SS
  Simulink-PS Converter3 : nesl_utility/Simulink-PS Converter  PhysicalDomain=network_engine_domain  SubClassName=ps_input  LeftPortType=input  RightPortType=output  PseudoPeriodic=off  Frequencies=[]  NoiseDistribution=none  NoiseParameters=[]  Unit=1  AffineConversion=off  FilteringAndDerivatives=provide  SimscapeFilterOrder=1  InputFilterTimeConstant=0.001  UdotUserProvided=0
      settings: SourceProductBaseCode=PW,SS
  Subsystem1 : Subsystem
  Unit Delay : UnitDelay  InitialCondition=-0.51*c_bar  SampleTime=-1  HasFrameUpgradeWarning=on
  left aero force and moment : MATLAB Function  TreatAsAtomicUnit=on
  xy in plane : sm_lib/Frames and Transforms/Rigid Transform  TranslationMethod=None  TranslationStandardOffset=0  TranslationLengthUnit=m  TranslationStandardAxis=+Z  TranslationCartesianOffset=[0 0 0]  TranslationROffset=0  TranslationROffsetUnits=m  TranslationZOffset=0  TranslationZOffsetUnits=m  TranslationThetaOffset=0  TranslationThetaOffsetUnits=deg  RotationMethod=RotationMatrix  RotationAngleUnits=deg  RotationStandardAxis=+Z  RotationAngle=0.0  RotationArbitraryAxis=[0 0 1]  FollAlignAxisA=+X  BaseAlignAxisA=+Y  FollAlignAxisB=+Y  BaseAlignAxisB=+Z  RotationSequenceAxes=FollowerAxes  RotationSequence=XYX  RotationSequenceAngles=[0 0 0]  RotationSequenceAnglesUnits=deg  RotationMatrix=[0 0 1; 0 -1 0; 1 0 0]
  W : PMIOPort  Side=Left
  WT : PMIOPort  Port=2  Side=Left
  CP : PMIOPort  Port=3  Side=Right
  Out Bus Element2 : Outport  PortName=left_rot  Element=b
  Out Bus Element1 : Outport  PortName=left_rot  Element=w
  Out Bus Element7 : Outport  PortName=left_rot  Element=q
  wires:
  PS-Simulink Converter14/1 -> [theta_l]
  PS-Simulink Converter1/1 -> [theta_dot_l]
  PS-Simulink Converter2/1 -> [theta_ddot_l]
  [theta_ddot_l] -> Out Bus Element2/1
  AoA/1(alpha) -> left aero force and moment/2(alpha)
  Subsystem1/1(le0) -> left aero force and moment/1(le0), AoA/1(le0)
  [theta_l] -> AoA/2(rot), Out Bus Element7/1
  [theta_dot_l] -> left aero force and moment/3(rot_dot), Out Bus Element1/1
  [r_cp] -> Simulink-PS Converter3/1
  [d_cp] -> Simulink-PS Converter2/1
  [M_rd] -> Simulink-PS Converter1/1
  [F_N] -> Simulink-PS Converter/1
  Constant/1 -> [r_cp]
  left aero force and moment/2(M_rd) -> Scope/2, [M_rd]
  left aero force and moment/1(F_N) -> Scope/1, [F_N]
  left aero force and moment/3(d_cp) -> Unit Delay/1
  Unit Delay/1 -> [d_cp]
  connections:
  External Force and Torque1/RConn1 -- xy in plane/LConn1 -- Revolute Joint/RConn1
  Revolute Joint/RConn2 -- PS-Simulink Converter14/LConn1
  Revolute Joint/RConn3 -- PS-Simulink Converter1/LConn1
  xy in plane/RConn1 -- File Solid/RConn1 -- Rectangular Joint/LConn1
  Simulink-PS Converter/RConn1 -- External Force and Torque/LConn2
  Simulink-PS Converter1/RConn1 -- External Force and Torque1/LConn1
  CP/RConn1 -- External Force and Torque/RConn1 -- Graphic/RConn1 -- Rectangular Joint/RConn1
  Revolute Joint/RConn4 -- PS-Simulink Converter2/LConn1
  WT/RConn1 -- Subsystem1/LConn2 -- Revolute Joint/LConn1
  W/RConn1 -- Subsystem1/LConn1
  Simulink-PS Converter2/RConn1 -- Rectangular Joint/LConn3
  Simulink-PS Converter3/RConn1 -- Rectangular Joint/LConn2
